simulink model "linear_model"  (R2016b)
settings: Solver=FixedStepAuto  StartTime=0.0  StopTime=1  FixedStep=0.02  RelTol=1e-3
values from neighbouring files (symbols this model uses):
  A = zeros(length(w), 5)    [leastSquare.m]    (also in leastSquare2.m = zeros(length(range), 4); read_id.m = fgets(S); testLinearPara.m = [  0 0 1)
  B = [0;C1;C2]    [testLinearPara.m]
  C = eye(3)    [testLinearPara.m]
  D = [0;0;0]    [testLinearPara.m]
  K = place(A, B, [-1 -2 -13])    [testLinearPara.m]
settings Model: Creator=Ernie  LastModifiedBy=Ernie

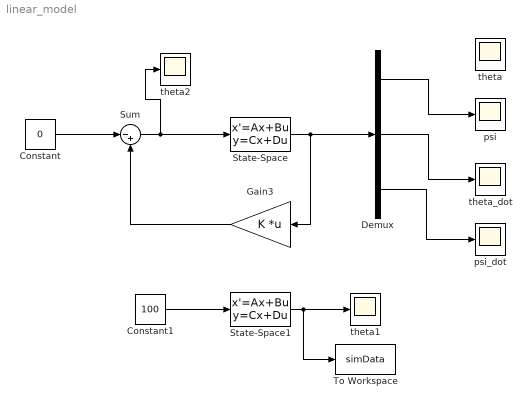
== system linear_model ==
  Constant : Constant  Value=0
  Constant1 : Constant  Value=100
  Demux : Demux  Outputs=3
  Gain3 : Gain  Gain=K  Multiplication=Matrix(K*u)
  State-Space : StateSpace  A=A  B=B  C=C  D=D  X0=[ 0.1745 0 0]
  State-Space1 : StateSpace  A=A  B=B  C=C  D=D  X0=[ 0.0 0 0]
  Sum : Sum  Inputs=|-+
  To Workspace : ToWorkspace  VariableName=simData  SaveFormat=Timeseries  SampleTime=-1
  psi : Scope
  psi_dot : Scope
  theta : Scope
  theta1 : Scope
  theta2 : Scope
  theta_dot : Scope
  wires:
  State-Space/1 -> Gain3/1, Demux/1
  Gain3/1 -> Sum/2
  Sum/1 -> theta2/1, State-Space/1
  Constant/1 -> Sum/1
  State-Space1/1 -> To Workspace/1, theta1/1
  Constant1/1 -> State-Space1/1
  Demux/1 -> psi/1
  Demux/2 -> theta_dot/1
  Demux/3 -> psi_dot/1
